simulink model "unza"  (R2014b)
settings: Solver=ode3  StartTime=0.0  StopTime=40  RelTol=1e-3
undefined symbols (not defined in the file or in its folder): frictionforce, g1, g2, g3, g4, mass, startspeed, stopspeed, unza
libraries: fuzblock x2
settings Model: Creator=linos_000  LastModifiedBy=linos_000
settings SolverCC: MaxConsecutiveMinStep=2  AutoInsertRateTranBlk=on

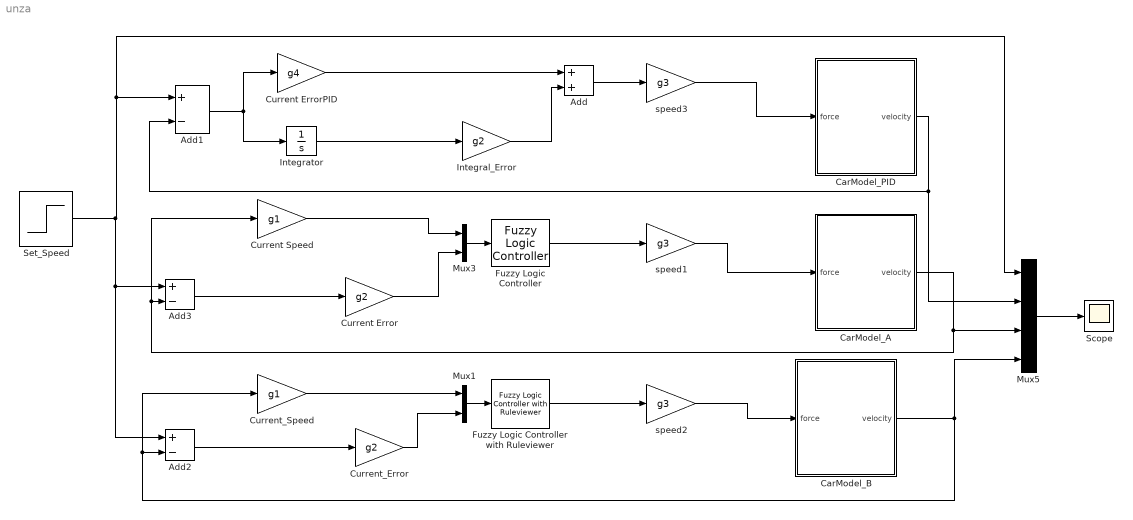
== system unza ==
  Add : Sum
  Add1 : Sum  Inputs=+-
  Add2 : Sum  Inputs=+-
  Add3 : Sum  Inputs=+-
  CarModel_A : Subsystem
  CarModel_B : Subsystem
  CarModel_PID : Subsystem
  Current Error : Gain  Gain=g2
  Current ErrorPID : Gain  Gain=g4
  Current Speed : Gain  Gain=g1
  Current_Error : Gain  Gain=g2
  Current_Speed : Gain  Gain=g1
  Fuzzy Logic Controller : fuzblock/Fuzzy Logic  Controller  fis=[unza]
  Fuzzy Logic Controller with Ruleviewer : fuzblock/Fuzzy Logic  Controller  with Ruleviewer  fismatrix=[unza]  Ts=2
  Integral_Error : Gain  Gain=g2
  Integrator : Integrator
  Mux1 : Mux  Inputs=2
  Mux3 : Mux  Inputs=2
  Mux5 : Mux
  Scope : Scope
      settings: ShowLegends=on  YMin=120  YMax=200
  Set_Speed : Step  Time=0  Before=startspeed  After=stopspeed  SampleTime=0
  speed1 : Gain  Gain=g3
  speed2 : Gain  Gain=g3
  speed3 : Gain  Gain=g3
  wires:
  Integral_Error/1 -> Add/2
  Current ErrorPID/1 -> Add/1
  Add1/1 -> Current ErrorPID/1, Integrator/1
  Integrator/1 -> Integral_Error/1
  CarModel_A/1(velocity) -> Mux5/3, Current Speed/1, Add3/2
  Current Error/1 -> Mux3/2
  Fuzzy Logic Controller/1 -> speed1/1
  Mux3/1 -> Fuzzy Logic Controller/1
  Current Speed/1 -> Mux3/1
  speed1/1 -> CarModel_A/1(force)
  Fuzzy Logic Controller with Ruleviewer/1 -> speed2/1
  Add2/1 -> Current_Error/1
  Add/1 -> speed3/1
  CarModel_B/1(velocity) -> Add2/2, Current_Speed/1, Mux5/4
  Current_Error/1 -> Mux1/2
  Current_Speed/1 -> Mux1/1
  Add3/1 -> Current Error/1
  Set_Speed/1 -> Mux5/1, Add1/1, Add2/1, Add3/1
  Mux5/1 -> Scope/1
  Mux1/1 -> Fuzzy Logic Controller with Ruleviewer/1
  speed2/1 -> CarModel_B/1(force)
  CarModel_PID/1(velocity) -> Add1/2, Mux5/2
  speed3/1 -> CarModel_PID/1(force)

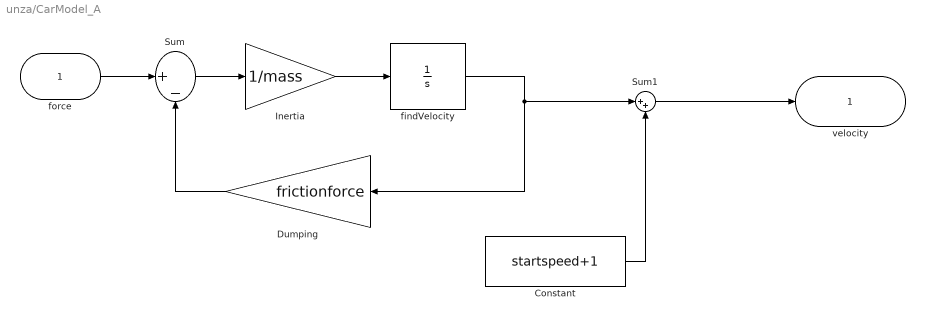
== system unza/CarModel_A ==
  force : Inport
  Constant : Constant  Value=startspeed+1
  Dumping : Gain  Gain=frictionforce
  Inertia : Gain  Gain=1/mass
  Sum : Sum  Inputs=|+-
  Sum1 : Sum  Inputs=|++
  findVelocity : Integrator
  velocity : Outport
  wires:
  findVelocity/1 -> Sum1/1, Dumping/1
  Inertia/1 -> findVelocity/1
  Dumping/1 -> Sum/2
  Sum/1 -> Inertia/1
  force/1 -> Sum/1
  Constant/1 -> Sum1/2
  Sum1/1 -> velocity/1

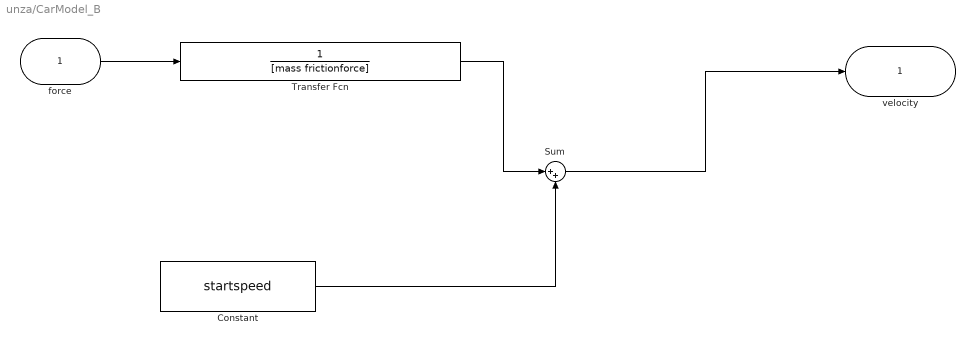
== system unza/CarModel_B ==
  force : Inport
  Constant : Constant  Value=startspeed
  Sum : Sum  Inputs=|++
  Transfer Fcn : TransferFcn  Denominator=[mass frictionforce]
  velocity : Outport
  wires:
  Constant/1 -> Sum/2
  force/1 -> Transfer Fcn/1
  Sum/1 -> velocity/1
  Transfer Fcn/1 -> Sum/1

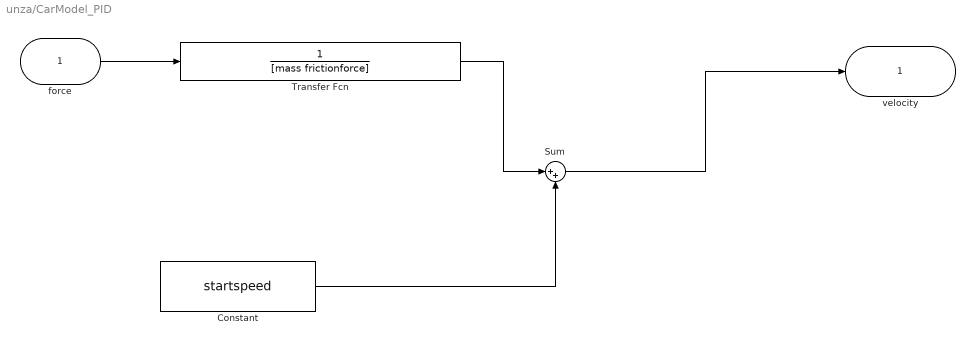
== system unza/CarModel_PID ==
  force : Inport
  Constant : Constant  Value=startspeed
  Sum : Sum  Inputs=|++
  Transfer Fcn : TransferFcn  Denominator=[mass frictionforce]
  velocity : Outport
  wires:
  Constant/1 -> Sum/2
  force/1 -> Transfer Fcn/1
  Sum/1 -> velocity/1
  Transfer Fcn/1 -> Sum/1
